simulink model "Controller"  (R2019b)
settings: Solver=VariableStepAuto  StartTime=0.0  StopTime=10.0  RelTol=1e-3
undefined symbols (not defined in the file): q0
settings Model: Creator=ariannagasparri  LastModifiedBy=ariannagasparri

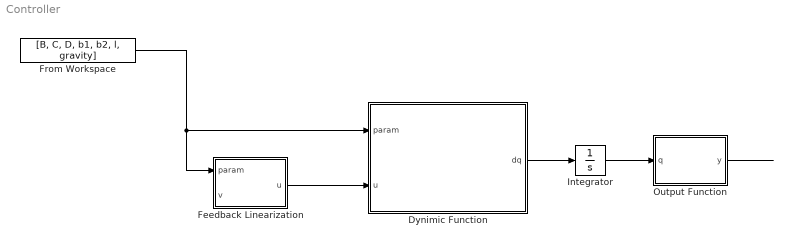
== system Controller ==
  Dynimic Function : MATLAB Function  TreatAsAtomicUnit=on
  Feedback Linearization : MATLAB Function  TreatAsAtomicUnit=on
  From Workspace : FromWorkspace  VariableName=[B, C, D, b1, b2, l, gravity]  SampleTime=0
  Integrator : Integrator  InitialCondition=q0
  Output Function : MATLAB Function  TreatAsAtomicUnit=on
  wires:
  Feedback Linearization/1(u) -> Dynimic Function/2(u)
  Dynimic Function/1(dq) -> Integrator/1
  Integrator/1 -> Output Function/1(q)
  Output Function/1(y) -> ?
  From Workspace/1 -> Feedback Linearization/1(param), Dynimic Function/1(param)

== matlab function Controller/Feedback Linearization ==
  data: param input; v input; u output
function u = fcn(param, v)

B = param(1);
C = param(2);
D = param(3);
b1 = param(4);
b2 = param(5);
l = param(6);
gravity = param(7);

u(1) = (v(1) - Lf2h1(B,C,D,b1,b2,gravity,l,q)) / LgLfh1(B,C,D,l,q);
u(2) = (v(2) - Lf2h2(B,C,b2,gravity,l,q)) / LgLfh2(B,C,D,l,q);

end

== matlab function Controller/Dynimic Function ==
  data: param input; u input; dq output
function dq = fcn(param, u)

B = param(1);
C = param(2);
D = param(3);
b1 = param(4);
b2 = param(5);
l = param(6);
gravity = param(7);

dq = f_fun(B,C,D,b1,b2,gravity,l,q) + g_fun(B,C,D,l,q)*u;

end

== matlab function Controller/Output Function ==
  data: q input; y output
function y = fcn(q)

y = h_fun(q);

end
